simulink model "Sim2LM2T"  (R2022b)
settings: Solver=VariableStepAuto  StartTime=0.0  StopTime=1000000  RelTol=1e-3
model workspace (MAT data in the model file):
  CuRRR50SH = 0.0994409039534
  r1 = 0.5
  r2 = 9.8
  steel304SH = 469.448840674
undefined symbols (not defined in the file or in its folder): Cold_T, Hot_T
libraries: fl_lib x14, nesl_utility x5
settings Model: Creator=andre.pianca  LastModifiedBy=andre.pianca

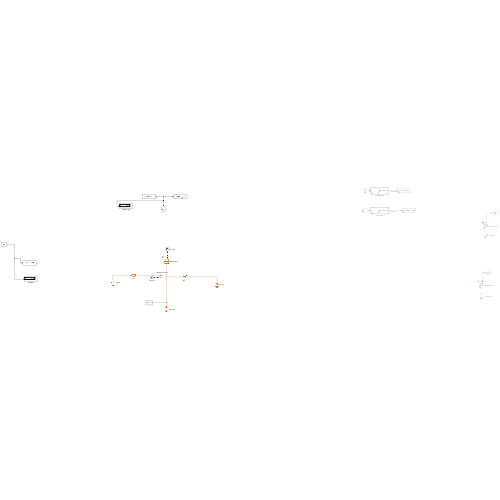
[thumbnail: Simulink's stored preview of the top-level diagram]
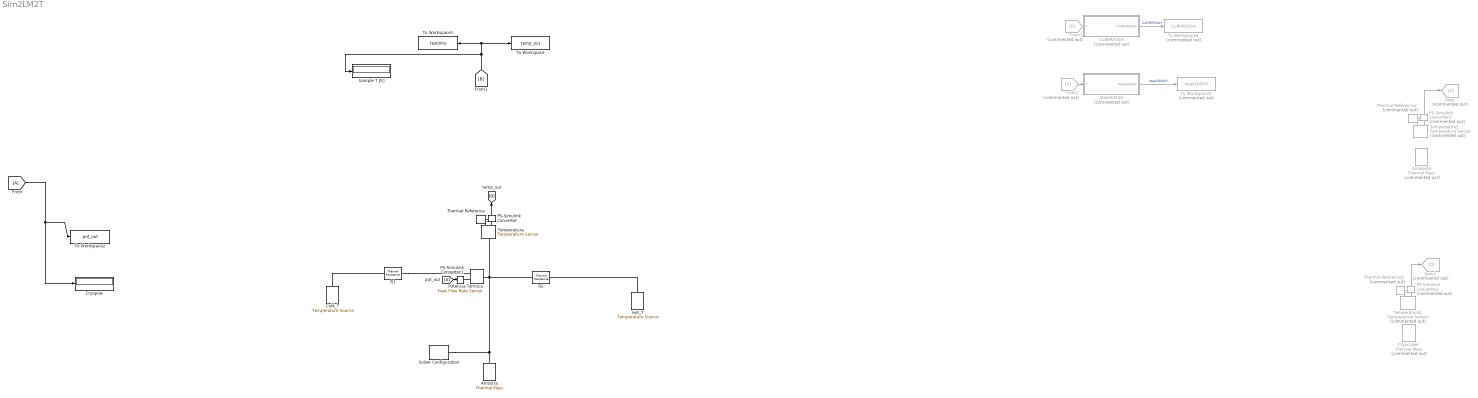
== system Sim2LM2T ==
  Ambiente : fl_lib/Thermal/Thermal Elements/Thermal Mass  Commented=on  mass=m_envsup kg  sp_heat=steel304SH J/(K*kg)  num_ports=foundation.enum.numPorts2.one  T_specify=on  T_priority=High  T=Hot_T K  T_nominal_specify=off  T_nominal_unit=K  T_nominal_value=1  Q_specify=off  Q_priority=None  Q=0 W  Q_nominal_specify=off  Q_nominal_unit=W  Q_nominal_value=1
  Amostra : fl_lib/Thermal/Thermal Elements/Thermal Mass  mass=m_sample kg  sp_heat=sh_sample J/(K*kg)  num_ports=foundation.enum.numPorts2.one  T_specify=off  T_priority=None  T=200 K  T_nominal_specify=off  T_nominal_unit=K  T_nominal_value=1  Q_specify=off  Q_priority=None  Q=0 W  Q_nominal_specify=off  Q_nominal_unit=W  Q_nominal_value=1
  Cold_T : fl_lib/Thermal/Thermal Sources/Temperature Source  temperature=Cold_T K
  Cryocooler : fl_lib/Thermal/Thermal Elements/Thermal Mass  Commented=on  mass=m_coldfing kg  sp_heat=CuRRR50SH J/(K*kg)  num_ports=foundation.enum.numPorts2.one  T_specify=on  T_priority=High  T=Cold_T K  T_nominal_specify=off  T_nominal_unit=K  T_nominal_value=1  Q_specify=off  Q_priority=None  Q=0 W  Q_nominal_specify=off  Q_nominal_unit=W  Q_nominal_value=1
  Cryopow : Display
  CuRRR50SH : MATLAB Function  Commented=on  TreatAsAtomicUnit=on
  From : From
  From2 : From  Commented=on  GotoTag=C
  From3 : From  Commented=on  GotoTag=D
  Goto : Goto  Commented=on  GotoTag=C
  Goto1 : Goto  Commented=on  GotoTag=D
  Hot_T : fl_lib/Thermal/Thermal Sources/Temperature Source  temperature=Hot_T K
  PS-Simulink Converter : nesl_utility/PS-Simulink Converter  PhysicalDomain=network_engine_domain  SubClassName=ps_output  LeftPortType=input  RightPortType=output  PseudoPeriodic=off  Frequencies=[]  VectorFormat=inherit  Unit=inherit  AffineConversion=off
  PS-Simulink Converter1 : nesl_utility/PS-Simulink Converter  PhysicalDomain=network_engine_domain  SubClassName=ps_output  LeftPortType=input  RightPortType=output  PseudoPeriodic=off  Frequencies=[]  VectorFormat=inherit  Unit=inherit  AffineConversion=off
  PS-Simulink Converter2 : nesl_utility/PS-Simulink Converter  Commented=on  PhysicalDomain=network_engine_domain  SubClassName=ps_output  LeftPortType=input  RightPortType=output  PseudoPeriodic=off  Frequencies=[]  VectorFormat=inherit  Unit=inherit  AffineConversion=off
  PS-Simulink Converter3 : nesl_utility/PS-Simulink Converter  Commented=on  PhysicalDomain=network_engine_domain  SubClassName=ps_output  LeftPortType=input  RightPortType=output  PseudoPeriodic=off  Frequencies=[]  VectorFormat=inherit  Unit=inherit  AffineConversion=off
  Potencia Termica : fl_lib/Thermal/Thermal Sensors/Heat Flow Rate Sensor
  R1 : fl_lib/Thermal/Thermal Elements/Thermal Resistance  resistance=r1_r K/W  T_specify=off  T_priority=None  T=0 K  T_nominal_specify=off  T_nominal_unit=K  T_nominal_value=1  Q_specify=off  Q_priority=None  Q=0 W  Q_nominal_specify=off  Q_nominal_unit=W  Q_nominal_value=1
  R2 : fl_lib/Thermal/Thermal Elements/Thermal Resistance  resistance=r2_r K/W  T_specify=off  T_priority=None  T=0 K  T_nominal_specify=off  T_nominal_unit=K  T_nominal_value=1  Q_specify=off  Q_priority=None  Q=0 W  Q_nominal_specify=off  Q_nominal_unit=W  Q_nominal_value=1
  Sample T [K] : Display
  Solver Configuration : nesl_utility/Solver Configuration  PhysicalDomain=network_engine_domain  SubClassName=solver  LeftPortType=input  RightPortType=generic  Tones=[]  Harmonics=[]  SimulateNoise=off  Profile=off  UseLocalSampling=off  EnableSwitchedLinearOptims=on  FrequencyDomain=off  UseCCode=off  RelTol=0.001  AbsTol=0.001  MinStep=1e-09  ToWorkspace=off  RevertToSquareIcSolve=off  NumHomotopyIterations=100  PhasorMode=off  PhasorModeNumHarmonics=1  ConsistencySolver=NEWTON_XTOL_AFTER_FTOL  IndexReductionMethod=DerivativeReplacement  DoDC=off  ResidualTolerance=1e-09  ConsistencyTolSource=GLOBAL  ConsistencyAbsTol=0.001  ConsistencyRelTol=0.001  ConsistencyTolFactor=0.001  UseLocalSolver=off  LocalSolverChoice=NE_BACKWARD_EULER_ADVANCER  ResolveIndetEquations=on  FunctionEvalNumThread=1  LocalSolverSampleTime=0.001  DoFixedCost=off  MaxNonlinIter=3  MaxModeIter=2  ComputeImpulses=off  ImpulseIterations=2  LinearAlgebra=auto  LinearAlgebraNumThread=0  EquationFormulation=NE_TIME_EF  DelaysMemoryBudget=1024  AutomaticFiltering=on  FilteringTimeConstant=0.001  PartitionStorageMethod=AS_NEEDED  PartitionMemoryBudget=1024  PartitionMethod=ROBUST
  Steel304SH : MATLAB Function  Commented=on  TreatAsAtomicUnit=on
  Temperatura : fl_lib/Thermal/Thermal Sensors/Temperature Sensor
  Temperatura1 : fl_lib/Thermal/Thermal Sensors/Temperature Sensor  Commented=on
  Temperatura2 : fl_lib/Thermal/Thermal Sensors/Temperature Sensor  Commented=on
  Thermal Reference : fl_lib/Thermal/Thermal Elements/Thermal Reference
  Thermal Reference1 : fl_lib/Thermal/Thermal Elements/Thermal Reference  Commented=on
  Thermal Reference2 : fl_lib/Thermal/Thermal Elements/Thermal Reference  Commented=on
  To Workspace : ToWorkspace  VariableName=temp_out  SampleTime=-1
      settings: Save2DSignal=2-D array (concatenate along first dimension)
  To Workspace1 : ToWorkspace  VariableName=testinho  SaveFormat=Timeseries  SampleTime=-1
      settings: Save2DSignal=2-D array (concatenate along first dimension)
  To Workspace2 : ToWorkspace  VariableName=pot_out  SampleTime=-1
      settings: Save2DSignal=2-D array (concatenate along first dimension)
  To Workspace4 : ToWorkspace  Commented=on  VariableName=CuRRR50SH  SaveFormat=Timeseries  SampleTime=-1
  To Workspace5 : ToWorkspace  Commented=on  VariableName=steel304SH  SaveFormat=Timeseries  SampleTime=-1
  pot_out : Goto
  wires:
  PS-Simulink Converter/1 -> [B]
  PS-Simulink Converter1/1 -> pot_out/1
  From/1 -> To Workspace2/1, Cryopow/1
  [B] -> Sample T [K]/1, To Workspace1/1, To Workspace/1
  CuRRR50SH/1(CuRRR50SH) -> To Workspace4/1  "CuRRR50SH"
  Steel304SH/1(steel304SH) -> To Workspace5/1  "steel304SH"
  From2/1 -> Steel304SH/1(T)
  PS-Simulink Converter3/1 -> Goto/1
  PS-Simulink Converter2/1 -> Goto1/1
  connections:
  Cold_T/LConn1 -- R1/LConn1
  Amostra/LConn1 -- Solver Configuration/RConn1 -- R2/LConn1 -- Potencia Termica/LConn1 -- Temperatura/LConn1
  Hot_T/LConn1 -- R2/RConn1
  Thermal Reference/LConn1 -- Temperatura/RConn1
  PS-Simulink Converter/LConn1 -- Temperatura/RConn2
  R1/RConn1 -- Potencia Termica/RConn2
  PS-Simulink Converter1/LConn1 -- Potencia Termica/RConn1
  Thermal Reference2/LConn1 -- Temperatura2/RConn1
  PS-Simulink Converter3/LConn1 -- Temperatura2/RConn2
  PS-Simulink Converter2/LConn1 -- Temperatura1/RConn2
  Thermal Reference1/LConn1 -- Temperatura1/RConn1

== matlab function Sim2LM2T/CuRRR50SH ==
  data: T input; CuRRR50SH output
function CuRRR50SH = fcn(T)

a = -1.91844;
b = -0.15973;
c = 8.61013;
d = -18.996;
e = 21.9661;
f = -12.7328;
g = 3.54322;
h = -0.3797;
i = 0;

CuRRR50SH = 10^(a+b*log10(T)+c*log10(T)^2+d*log10(T)^3+e*log10(T)^4+f*log10(T)^5+g*log10(T)^6+h*log10(T)^7+i*log10(T)^8);

== matlab function Sim2LM2T/Steel304SH ==
  data: T input; steel304SH output
function steel304SH = fcn(T)

a = 22.0061;
b = -127.5528;
c = 303.647;
d = -381.0098;
e = 274.0328;
f = -112.9212;
g = 24.7593;
h = -2.239153;
i = 0;



steel304SH = 10^(a+b*log10(T)+c*log10(T)^2+d*log10(T)^3+e*log10(T)^4+f*log10(T)^5+g*log10(T)^6+h*log10(T)^7+i*log10(T)^8);
